simulink model "csu_kir_image_request_hrn"  (R2014b)
settings: Solver=FixedStepDiscrete  StartTime=0.0  StopTime=1  FixedStep=1  RelTol=1e-3
libraries: csu_kir_image_request_lib x1
settings Model: Creator=escrane  LastModifiedBy=mstewart
settings DebuggingCC: UnderspecifiedInitializationDetection=Classic  MergeDetectMultiDrivingBlocksExec=none  StateNameClashWarn=warning

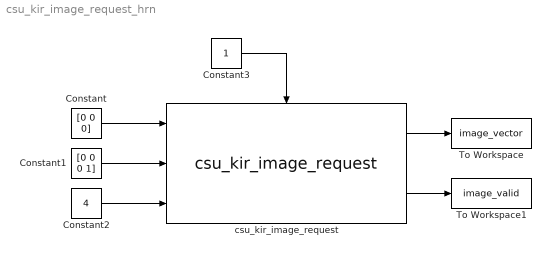
== system csu_kir_image_request_hrn ==
  Constant : Constant  Value=[0 0 0]
  Constant1 : Constant  Value=[0 0 0 1]
  Constant2 : Constant  Value=4
  Constant3 : Constant
  To Workspace : ToWorkspace  VariableName=image_vector  SaveFormat=Timeseries  SampleTime=-1
  To Workspace1 : ToWorkspace  VariableName=image_valid  SaveFormat=Timeseries  SampleTime=-1
  csu_kir_image_request : csu_kir_image_request_lib/csu_kir_image_request  size=cam_kir_image_size  intrinsics=cam_kir_intrinsics
  wires:
  Constant/1 -> csu_kir_image_request/1
  Constant1/1 -> csu_kir_image_request/2
  Constant2/1 -> csu_kir_image_request/3
  csu_kir_image_request/1 -> To Workspace/1
  csu_kir_image_request/2 -> To Workspace1/1
  Constant3/1 -> csu_kir_image_request/Enable
